simulink library "fixpt_megmalib"  (Simulink 6.0)
settings: Solver=ode45  SolverMode=SingleTasking  StartTime=0.0  StopTime=10.0  RelTol=1e-3
undefined symbols (not defined in the file or in its folder): Bias1, Bias2, NumBits1, NumBits2, Slope1, Slope2
libraries: simulink x94, fixpt_megmaFuncBlkhidden1 x5, fixpt_megmalib x3
(part 3 of 3)

== system fixpt_megmalib/Low and Highpass/LowPass TResetEnabled/ResetEnabledState ==
  E : Inport  LatchInput=off
  R : Inport  Port=2  LatchInput=off
  IV : Inport  Port=3  LatchInput=off
  Xcalc : Inport  Port=4  LatchInput=off
  Unit Delay With Preview Enabled Resettable External RV : simulink/Additional Math & Discrete/Additional Discrete/Unit Delay With Preview Enabled Resettable External RV  vinit=0.0  tsamp=-1
  Xnew : Outport
  Xold : Outport  Port=2
  wires:
  Unit Delay With Preview Enabled Resettable External RV/2 -> Xold/1
  Unit Delay With Preview Enabled Resettable External RV/1 -> Xnew/1
  IV/1 -> Unit Delay With Preview Enabled Resettable External RV/4
  R/1 -> Unit Delay With Preview Enabled Resettable External RV/3
  E/1 -> Unit Delay With Preview Enabled Resettable External RV/2
  Xcalc/1 -> Unit Delay With Preview Enabled Resettable External RV/1

== system fixpt_megmalib/Nonlinear Blocks/MeanValue/ResetEnabledTappedDelay ==
  E : Inport  LatchInput=off
  R : Inport  Port=2  LatchInput=off
  IV : Inport  Port=3  LatchInput=off
  u : Inport  Port=4  LatchInput=off
  FixPt Data Type Duplicate1 : simulink/Signal Attributes/Data Type Duplicate  NumInputPorts=5
  FixPt Switch1 : Switch  Threshold=1  ZeroCross=off
  FixPt Switch3 : Switch  Threshold=1  ZeroCross=off
  FixPt Unit Delay1 : UnitDelay  X0=0.0  SampleTime=-1
  Mux : Mux  Inputs=2
  Selector : Selector  Orientation=left  Elements=1:(nSample-1)  InputPortWidth=nSample
  Xnew : Outport
  wires:
  Mux/1 -> FixPt Switch3/1
  Selector/1 -> Mux/2
  u/1 -> FixPt Data Type Duplicate1/5, Mux/1
  R/1 -> FixPt Switch1/2  "Reset"
  FixPt Switch1/1 -> FixPt Unit Delay1/1, FixPt Data Type Duplicate1/2, Xnew/1  "Xnew"
  FixPt Unit Delay1/1 -> Selector/1, FixPt Switch3/3, FixPt Data Type Duplicate1/1  "Xold"
  FixPt Switch3/1 -> FixPt Switch1/3, FixPt Data Type Duplicate1/4
  IV/1 -> FixPt Switch1/1, FixPt Data Type Duplicate1/3  "Initial Value"
  E/1 -> FixPt Switch3/2  "Enable"
